simulink model "Accelerometer_R2023a"  (R2023a)
settings: Solver=ode4  StartTime=0.0  StopTime=10  FixedStep=sim.dt  RelTol=1e-3
undefined symbols (not defined in the file or in its folder): a_bias, a_sath, a_satl, a_sf_cc, acc, fin_maxrate, sim
libraries: aerolibnav x3, aerolibcommonsys x2, mspsensorlib x1, sharedutil x1
settings Model: Creator=mhcho  LastModifiedBy=mhcho
settings DebuggingCC: UnconnectedInputMsg=warning  UnconnectedOutputMsg=warning  UnconnectedLineMsg=warning
settings ModelReferenceCC: EnableRefExpFcnMdlSchedulingChecks=on
settings RTWCC: DLArmComputeVersion=19.05

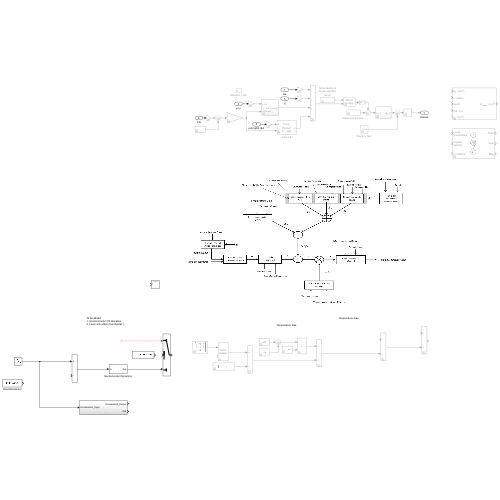
[thumbnail: Simulink's stored preview of the top-level diagram]
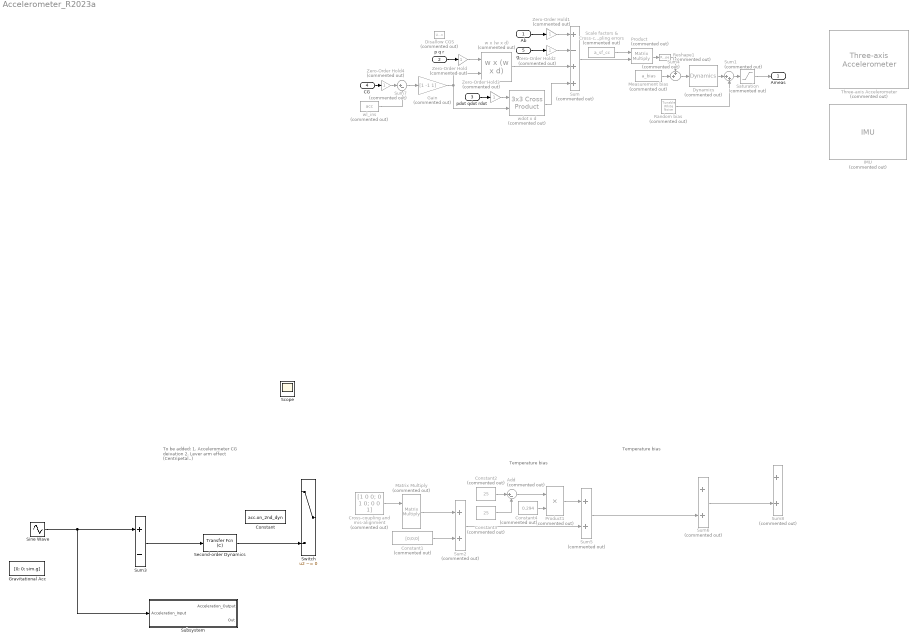
== system Accelerometer_R2023a ==
  note: Temperature bias
  note: To be added:
      | 1. Accelerometer CG deivation
      | 2. Lever arm effect (Centripetal..)
  note: Temperature bias
  Ab : Inport  Unit=m/s^2  PortDimensions=3
  p q r : Inport  Port=2  Unit=rad/s  PortDimensions=3
  pdot qdot rdot : Inport  Port=3  Unit=rad/s^2  PortDimensions=3
  CG : Inport  Port=4  Unit=m  PortDimensions=3
  g : Inport  Port=5  Unit=m/s^2  PortDimensions=3
  Add : Sum  Commented=on  Inputs=|+-
  Constant : Constant  Value=acc.on_2nd_dyn
  Constant1 : Constant  Commented=on  Value=[0;0;0]
  Constant2 : Constant  Commented=on  Value=25
  Constant3 : Constant  Commented=on  Value=25
  Constant4 : Constant  Commented=on  Value=0.294
  Cross-coupling and mis-alignment : Constant  Commented=on  Value=[1 0 0; 0 1 0; 0 0 1]
  Disallow CGS : UnitConfiguration  Commented=on  UnitSystemsStr=English,SI,SI (extended)  AllowAllUnitSystems=off
  Dynamics : aerolibnav/Three-axis Accelerometer/Dynamics  Commented=on  SystemSampleTime=-1  VariantActivationTime=update diagram  Latency=0  AutoFrameSizeCalculation=off
  Gain : Gain  Commented=on  Gain=[1 -1 1]  SaturateOnIntegerOverflow=on  OutDataTypeStr=Inherit: Same as input  ParamDataTypeStr=Inherit: Same as input
  Gravitational Acc : Constant  Value=[0; 0; sim.g]
  IMU : mspsensorlib/IMU  Commented=on  DispRefFrame=NED  Temperature=25  MagneticFieldNED=[ 27.5550, -2.4169, -16.0849 ]  MagneticFieldENU=[ -2.4169, 27.5550, 16.0849 ]  SeedDouble=67  SimulateUsing=Interpreted execution  AccelParamsMeasurementRange=Inf  AccelParamsResolution=0  AccelParamsConstantBias=[ 0, 0, 0 ]  AccelParamsAxesMisalignment=[ 0, 0, 0 ]  AccelParamsNoiseDensity=[ 0, 0, 0 ]  AccelParamsBiasInstability=[ 0, 0, 0 ]  AccelParamsRandomWalk=[ 0, 0, 0 ]  AccelParamsTemperatureBias=[ 0, 0, 0 ]  AccelParamsTemperatureScaleFactor=[ 0, 0, 0 ]  GyroParamsMeasurementRange=Inf  GyroParamsResolution=0  GyroParamsConstantBias=[ 0, 0, 0 ]  GyroParamsAxesMisalignment=[ 0, 0, 0 ]  GyroParamsAccelerationBias=[ 0, 0, 0 ]  GyroParamsNoiseDensity=[ 0, 0, 0 ]  GyroParamsBiasInstability=[ 0, 0, 0 ]  GyroParamsRandomWalk=[ 0, 0, 0 ]  GyroParamsTemperatureBias=[ 0, 0, 0 ]  GyroParamsTemperatureScaleFactor=[ 0, 0, 0 ]  MagParamsMeasurementRange=Inf  MagParamsResolution=0  MagParamsConstantBias=[ 0, 0, 0 ]  MagParamsAxesMisalignment=[ 0, 0, 0 ]  MagParamsNoiseDensity=[ 0, 0, 0 ]  MagParamsBiasInstability=[ 0, 0, 0 ]  MagParamsRandomWalk=[ 0, 0, 0 ]  MagParamsTemperatureBias=[ 0, 0, 0 ]  MagParamsTemperatureScaleFactor=[ 0, 0, 0 ]
  Matrix Multiply : Product  Commented=on  Multiplication=Matrix(*)
  Measurement bias : Constant  Commented=on  Value=a_bias
  Product : Product  Commented=on  Multiplication=Matrix(*)  SaturateOnIntegerOverflow=on  OutDataTypeStr=Inherit: Same as first input
  Product1 : Product  Commented=on
  Random bias : aerolibcommonsys/Tunable White Noise  Commented=on  pwr=a_pow  Ts=0.1  seed=a_seeds
  Reshape1 : Reshape  Commented=on
  Saturation : Saturate  Commented=on  UpperLimit=a_sath  LowerLimit=a_satl
  Scale factors & Cross-coupling errors : Constant  Commented=on  Value=a_sf_cc
  Scope : Scope
  Second-order Dynamics : aerolibcommonsys/Transfer Fcn (C)  wn=sqrt(acc.stiffness/acc.mass_proof)  zn=acc.damping/(2*sqrt(acc.stiffness*acc.mass_proof))
  Sine Wave : Sin  Frequency=2*pi
  Subsystem : Subsystem
  Sum : Sum  Commented=on  Inputs=+-++  SaturateOnIntegerOverflow=on
  Sum1 : Sum  Commented=on  Inputs=|++  SaturateOnIntegerOverflow=on
  Sum{2,5..6,8} (4 alike) : Sum  Commented=on
  Sum3 : Sum  Inputs=+-
  Sum4 : Sum  Commented=on  Inputs=++|  SaturateOnIntegerOverflow=on
  Sum7 : Sum  Commented=on  Inputs=|+-  SaturateOnIntegerOverflow=on
  Switch : Switch  Criteria=u2 ~= 0  Threshold=0.5  SaturateOnIntegerOverflow=off  InputSameDT=off
  Three-axis Accelerometer : aerolibnav/Three-axis Accelerometer  Commented=on  units=Metric (MKS)  acc=[0 0 0]  gtype=on  dtype_a=on  w_a=190  z_a=0.707  a_sf_cc=[1 0 0; 0 1 0; 0 0 1]  a_bias=[0 0 0]  a_Ts=0  a_rand=on  a_seeds=[23093 23094 23095]  a_pow=[0.001 0.001 0.001]  a_sat="[-inf  -inf  -inf  inf inf inf]"
  Zero-Order Hold{,1..4} (5 alike) : Gain  Commented=on  SaturateOnIntegerOverflow=on  OutDataTypeStr=Inherit: Same as input  ParamDataTypeStr=Inherit: Same as input
  w x (w x d) : aerolibnav/Three-axis Accelerometer/w x (w x d)  Commented=on  SystemSampleTime=-1  VariantActivationTime=update diagram  Latency=0  AutoFrameSizeCalculation=off
  wdot x d : sharedutil/3x3 Cross Product  Commented=on  aMode=aMode
  wl_ins : Constant  Commented=on  Value=acc
  Ameas : Outport  Unit=m/s^2  PortDimensions=3  VectorParamsAs1DForOutWhenUnconnected=off
  wires:
  Sum/1 -> Product/2
  Saturation/1 -> Ameas/1
  Scale factors & Cross-coupling errors/1 -> Product/1
  Zero-Order Hold1/1 -> Sum/1
  Sum4/1 -> Dynamics/1
  Gain/1 -> wdot x d/2, w x (w x d)/2
  p q r/1 -> Zero-Order Hold/1
  wdot x d/1 -> Sum/4
  CG/1 -> Zero-Order Hold4/1
  Random bias/1 -> Sum1/2
  Measurement bias/1 -> Sum4/2
  Ab/1 -> Zero-Order Hold1/1
  Sum7/1 -> Gain/1
  w x (w x d)/1 -> Sum/3
  Zero-Order Hold4/1 -> Sum7/1
  Sum1/1 -> Saturation/1
  Zero-Order Hold/1 -> w x (w x d)/1
  g/1 -> Zero-Order Hold2/1
  Reshape1/1 -> Sum4/1
  Zero-Order Hold3/1 -> wdot x d/1
  pdot qdot rdot/1 -> Zero-Order Hold3/1
  Dynamics/1 -> Sum1/1
  Zero-Order Hold2/1 -> Sum/2
  Product/1 -> Reshape1/1
  wl_ins/1 -> Sum7/2
  ? -> Switch/1
  Sine Wave/1 -> Subsystem/1(Acceleration_Input), Sum3/1
  Sum3/1 -> Second-order Dynamics/1
  Cross-coupling and mis-alignment/1 -> Matrix Multiply/1
  Matrix Multiply/1 -> Sum2/1
  Constant1/1 -> Sum2/2
  Sum2/1 -> Sum5/2
  Product1/1 -> Sum5/1
  Add/1 -> Product1/1
  Constant2/1 -> Add/1
  Constant3/1 -> Add/2
  Constant4/1 -> Product1/2
  Sum5/1 -> Sum6/2
  Sum6/1 -> Sum8/2
  Second-order Dynamics/1 -> Switch/3

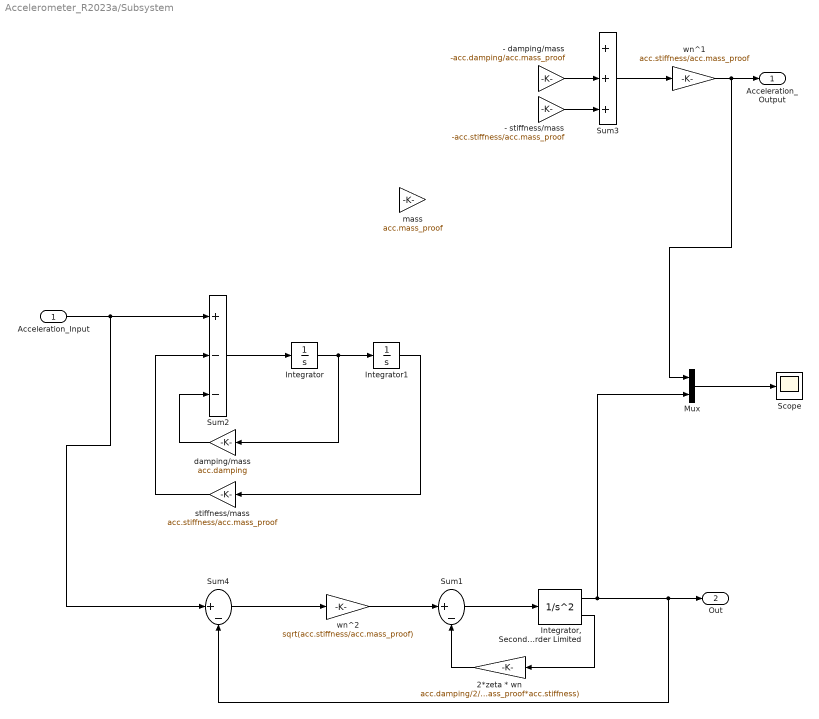
== system Accelerometer_R2023a/Subsystem ==
  Acceleration_Input : Inport
  - damping/mass : Gain  Gain=-acc.damping/acc.mass_proof
  - stiffness/mass : Gain  Gain=-acc.stiffness/acc.mass_proof
  2*zeta * wn : Gain  Gain=acc.damping/2/sqrt(acc.mass_proof*acc.stiffness)  SaturateOnIntegerOverflow=on  OutDataTypeStr=Inherit: Same as input  ParamDataTypeStr=Inherit: Same as input
  Integrator : Integrator
  "Integrator, Second-Order Limited" : SecondOrderIntegrator  ICX=0  UpperLimitX=fin_max  LowerLimitX=fin_min  ICDXDT=0  UpperLimitDXDT=fin_maxrate  LowerLimitDXDT=-fin_maxrate
  Integrator1 : Integrator
  Mux : Mux  Inputs=2
  Scope : Scope
  Sum1 : Sum  Inputs=|+-  InputSameDT=on  SaturateOnIntegerOverflow=on  OutDataTypeStr=Inherit: Same as first input
  Sum2 : Sum  Inputs=+--  SaturateOnIntegerOverflow=on
  Sum3 : Sum  Inputs=+++
  Sum4 : Sum  Inputs=|+-  InputSameDT=on  SaturateOnIntegerOverflow=on  OutDataTypeStr=Inherit: Same as first input
  damping/mass : Gain  Gain=acc.damping
  mass : Gain  Gain=acc.mass_proof
  stiffness/mass : Gain  Gain=acc.stiffness/acc.mass_proof
  wn^1 : Gain  Gain=acc.stiffness/acc.mass_proof  SaturateOnIntegerOverflow=on  OutDataTypeStr=Inherit: Same as input  ParamDataTypeStr=Inherit: Same as input
  wn^2 : Gain  Gain=sqrt(acc.stiffness/acc.mass_proof)  SaturateOnIntegerOverflow=on  OutDataTypeStr=Inherit: Same as input  ParamDataTypeStr=Inherit: Same as input
  Acceleration_Output : Outport
  Out : Outport  Port=2  VectorParamsAs1DForOutWhenUnconnected=off
  wires:
  Sum2/1 -> Integrator/1
  Integrator/1 -> Integrator1/1, damping/mass/1
  Integrator1/1 -> stiffness/mass/1
  damping/mass/1 -> Sum2/3
  stiffness/mass/1 -> Sum2/2
  - damping/mass/1 -> Sum3/2
  - stiffness/mass/1 -> Sum3/3
  Sum3/1 -> wn^1/1
  wn^2/1 -> Sum1/1
  "Integrator, Second-Order Limited"/2 -> 2*zeta * wn/1
  "Integrator, Second-Order Limited"/1 -> Out/1, Sum4/2, Mux/2
  2*zeta * wn/1 -> Sum1/2
  Sum4/1 -> wn^2/1
  Acceleration_Input/1 -> Sum4/1, Sum2/1
  Sum1/1 -> "Integrator, Second-Order Limited"/1
  Mux/1 -> Scope/1
  wn^1/1 -> Mux/1, Acceleration_Output/1
